simulink model "PID_reference_Q4W2"  (R2020b)
settings: Solver=VariableStepAuto  StartTime=0.0  StopTime=10.0  RelTol=1e-3
values from neighbouring files (symbols this model uses):
  Kd = 1.0    [DataDict_PID_Q4W2.sldd]    (also in W2ques4_code.m = 0.15)
  Ki = 1.0    [DataDict_PID_Q4W2.sldd]    (also in W2ques4_code.m = 500)
  Kp = 1.0    [DataDict_PID_Q4W2.sldd]    (also in W2ques4_code.m = 21)
settings Model: DataDictionary=DataDict_PID_Q4W2.sldd  EnableAccessToBaseWorkspace=off  Creator=sneha  LastModifiedBy=sneha
settings DataIOCC: SaveOutput=off  SaveTime=off

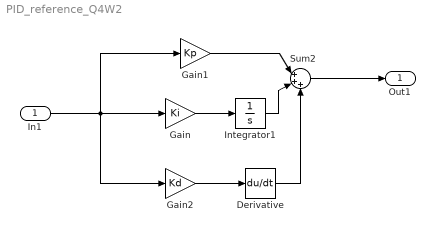
== system PID_reference_Q4W2 ==
  In1 : Inport  OutDataTypeStr=double  PortDimensions=1  SampleTime=0
  Derivative : Derivative
  Gain : Gain  Gain=Ki
  Gain1 : Gain  Gain=Kp
  Gain2 : Gain  Gain=Kd
  Integrator1 : Integrator
  Sum2 : Sum  Inputs=|+++
  Out1 : Outport  OutDataTypeStr=double  PortDimensions=1  SampleTime=0
  wires:
  Gain1/1 -> Sum2/1
  In1/1 -> Gain/1, Gain1/1, Gain2/1
  Derivative/1 -> Sum2/3
  Integrator1/1 -> Sum2/2
  Sum2/1 -> Out1/1
  Gain/1 -> Integrator1/1
  Gain2/1 -> Derivative/1
